simulink model "VCU_SW_1"  (R2023b)
settings: Solver=FixedStepDiscrete  StartTime=0.0  StopTime=inf  FixedStep=1e-2  RelTol=1e-3
PreLoadFcn:
  | RTWConfigurationCB('preloadfcn', bdroot);
InitFcn:
  | loadvar_ttc500
undefined symbols (not defined in the file): BrkPedalTypes, CabMovModeTypes, cFuseTempSensAcc_X, cFuseTempSensAcc_Y, cFuseTempSensVal_X, cFuseTempSensVal_Y, cTMSTempSensVal_X, cTMSTempSensVal_Y, cTransferCaseSpeedRatio, diag_state, DoorsPositionTypes, dP_filter_Y, DriverOccClassSystemTypes, ErrorValueTypes, fatal_error_callback, IO_ADC_NO_RANGE, LadderStatusTypes, pAnalogCabRotSensAcc, pAnalogCabRotSensMaxVolt, pAnalogCabRotSensMinVolt, pAnalogCabRotSensRange, pAnalogCabRotSensZeroVolt, pBrkActivePress, pCabTiltSensAcc, pCabTiltSensMaxCur, pCabTiltSensMinCur, pDistanceCorrection, pECANManual_BPNEnable, pECANManual_BPNEnabler_Flag, pFilterSensAccRes, pHDirMaxDiffFrq, pHDirSensHighLvl, pHDirSensLowLvl, pMainGearRatio, pMaxFilterSensRes, pMaxFirstPedalSensValue, pMaxFuseTempSensRes, pMaxPressLoss, pMaxPressSensCurrent, pMaxPressValue, pMaxPressValueHydMotAndPump, pMaxPressValueParkDrain, pMaxSecondPedalSensValue, pMaxTempSensVoltage, pMaxTempValue, pMaxTMSTempSensRes, pMinFilterSensRes, pMinFirstPedalSensValue, pMinFuseTempSensRes, pMinPressLoss, pMinPressSensCurrent, pMinPressValue, pMinSecondPedalSensValue, pMinTempSensVoltage, pMinTempValue, pMinTMSTempSensRes, pMotorRingTeethNum, pPedalSensAccuracyPct, pPedalSensAccuracyVolt, pPressLossTreshhold ... (+20)
libraries: TTlibrary x270, canmsglib x127, simulink x88
(part 4 of 19)

== system VCU_SW_1/InputLayer/InputInterfaces/PWDInput/GetPWD100msec ==
  function : TriggerPort  TriggerType=function-call  VariantControl=Variant
  Bus Selector : BusSelector  OutputSignals=pulse_samples_count
  Bus Selector1 : BusSelector  OutputSignals=pulse_samples_count
  Data Store Write : DataStoreWrite  DataStoreName=LogInputInterfaceData  DataStoreElements=LogInputInterfaceData.AI_1_Log.log_transPumpSpdSensSig2  IndexOptions=Index vector (dialog)  Indices=1  OutputSizes=1
  Data Store Write1 : DataStoreWrite  DataStoreName=InputInterfaceData  DataStoreElements=InputInterfaceData.PWD.transmHydMotSpdSensSig1  IndexOptions=Index vector (dialog)  Indices=1  OutputSizes=1
  Data Store Write10 : DataStoreWrite  DataStoreName=UDSStruct  DataStoreElements=UDSStruct.pin_transmHydMotSpdSensSig1  IndexOptions=Index vector (dialog)  Indices=1  OutputSizes=1
  Data Store Write11 : DataStoreWrite  DataStoreName=UDSStruct  DataStoreElements=UDSStruct.pin_transmHydMotSpdSensSig2  IndexOptions=Index vector (dialog)  Indices=1  OutputSizes=1
  Data Store Write12 : DataStoreWrite  DataStoreName=UDSStruct  DataStoreElements=UDSStruct.pin_transPumpSpdSensSig2  IndexOptions=Index vector (dialog)  Indices=1  OutputSizes=1
  Data Store Write13 : DataStoreWrite  DataStoreName=UDSStruct  DataStoreElements=UDSStruct.pin_transPumpSpdSensSig1  IndexOptions=Index vector (dialog)  Indices=1  OutputSizes=1
  Data Store Write2 : DataStoreWrite  DataStoreName=InputInterfaceData  DataStoreElements=InputInterfaceData.PWD.transmHydMotSpdSensSig2  IndexOptions=Index vector (dialog)  Indices=1  OutputSizes=1
  Data Store Write3 : DataStoreWrite  DataStoreName=InputInterfaceData  DataStoreElements=InputInterfaceData.PWD.transPumpSpdSensSig2  IndexOptions=Index vector (dialog)  Indices=1  OutputSizes=1
  Data Store Write4 : DataStoreWrite  DataStoreName=InputInterfaceData  DataStoreElements=InputInterfaceData.PWD.transPumpSpdSensSig1  IndexOptions=Index vector (dialog)  Indices=1  OutputSizes=1
  Data Store Write5 : DataStoreWrite  DataStoreName=LogInputInterfaceData  DataStoreElements=LogInputInterfaceData.AI_1_Log.log_transPumpSpdSensSig1  IndexOptions=Index vector (dialog)  Indices=1  OutputSizes=1
  Data Store Write6 : DataStoreWrite  DataStoreName=LogInputInterfaceData  DataStoreElements=LogInputInterfaceData.AI_2_Log.log_transmHydMotSpdSensSig1  IndexOptions=Index vector (dialog)  Indices=1  OutputSizes=1
  Data Store Write7 : DataStoreWrite  DataStoreName=LogInputInterfaceData  DataStoreElements=LogInputInterfaceData.AI_2_Log.log_transmHydMotSpdSensSig2  IndexOptions=Index vector (dialog)  Indices=1  OutputSizes=1
  Data Store Write8 : DataStoreWrite  DataStoreName=InputInterfaceData  DataStoreElements=InputInterfaceData.PWD.transmHydMotPulseSamples1  IndexOptions=Index vector (dialog)  Indices=1  OutputSizes=1
  Data Store Write9 : DataStoreWrite  DataStoreName=InputInterfaceData  DataStoreElements=InputInterfaceData.PWD.transmHydMotPulseSamples2  IndexOptions=Index vector (dialog)  Indices=1  OutputSizes=1
  Data Type Conversion : DataTypeConversion  OutDataTypeStr=uint16  SaturateOnIntegerOverflow=off  RndMeth=Floor
  Data Type Conversion1 : DataTypeConversion  OutDataTypeStr=uint16  SaturateOnIntegerOverflow=off  RndMeth=Floor
  Function Caller{,1..3} (4 alike) : FunctionCaller  FunctionPrototype=finalValue = convPWDData(rawValue,errorSts)  InputArgumentSpecifications=<Enter example>  OutputArgumentSpecifications=<Enter example>
  MATLAB Function8 : MATLAB Function  Commented=on  TreatAsAtomicUnit=on
  Terminator{,1..4,6,8..10,12} (10 alike) : Terminator
  TransPumpSpeedSensSig1 : TTlibrary/PWD/pwdComplexGet  timer_channel=IO_PWD_01  pulse_mode=IO_PWD_HIGH_TIME  freq_mode=IO_PWD_RISING_VAR  capture_count=4  pupd=IO_PWD_PD_10K  safety_conf=off  pwd_freq_val_lower=0  pwd_freq_val_upper=0  pwd_pulse_val_lower=0  pwd_pulse_val_upper=0  io_error=on  sample_time=-1
      settings: SourceProductName=TT control 500 series
  TransPumpSpeedSensSig2 : TTlibrary/PWD/pwdComplexGet  timer_channel=IO_PWD_03  pulse_mode=IO_PWD_HIGH_TIME  freq_mode=IO_PWD_RISING_VAR  capture_count=4  pupd=IO_PWD_PD_10K  safety_conf=off  pwd_freq_val_lower=0  pwd_freq_val_upper=0  pwd_pulse_val_lower=0  pwd_pulse_val_upper=0  io_error=on  sample_time=-1
      settings: SourceProductName=TT control 500 series
  TransmHydromotorSpeedAndPulseSig1 : TTlibrary/PWD/pwdComplexGet  timer_channel=IO_PWD_02  pulse_mode=IO_PWD_HIGH_TIME  freq_mode=IO_PWD_RISING_VAR  capture_count=4  pupd=IO_PWD_PD_10K  safety_conf=off  pwd_freq_val_lower=0  pwd_freq_val_upper=0  pwd_pulse_val_lower=0  pwd_pulse_val_upper=0  io_error=on  sample_time=-1
      settings: SourceProductName=TT control 500 series
  TransmHydromotorSpeedAndPulseSig2 : TTlibrary/PWD/pwdComplexGet  timer_channel=IO_PWD_04  pulse_mode=IO_PWD_HIGH_TIME  freq_mode=IO_PWD_RISING_VAR  capture_count=4  pupd=IO_PWD_PD_10K  safety_conf=off  pwd_freq_val_lower=0  pwd_freq_val_upper=0  pwd_pulse_val_lower=0  pwd_pulse_val_upper=0  io_error=on  sample_time=-1
      settings: SourceProductName=TT control 500 series
  wires:
  Data Type Conversion1/1 -> Data Store Write9/1
  TransmHydromotorSpeedAndPulseSig2/4 -> Bus Selector1/1  "io_pwd_04_samples"
  Bus Selector1/1 -> Data Type Conversion1/1  "<pulse_samples_count>"
  Data Type Conversion/1 -> Data Store Write8/1
  Bus Selector/1 -> Data Type Conversion/1  "<pulse_samples_count>"
  TransmHydromotorSpeedAndPulseSig1/4 -> Bus Selector/1  "io_pwd_02_samples"
  TransmHydromotorSpeedAndPulseSig2/1 -> Function Caller1/1  "io_pwd_04_freq_value"
  TransPumpSpeedSensSig2/1 -> Function Caller3/1  "io_pwd_03_freq_value"
  TransPumpSpeedSensSig1/1 -> Function Caller2/1  "io_pwd_01_freq_value"
  TransPumpSpeedSensSig2/4 -> Terminator10/1  "io_pwd_03_samples"
  TransPumpSpeedSensSig2/3 -> Terminator4/1  "io_pwd_03_pin_value"
  Function Caller/1 -> Data Store Write6/1, Data Store Write1/1
  TransPumpSpeedSensSig1/4 -> Terminator8/1  "io_pwd_01_samples"
  TransPumpSpeedSensSig2/2 -> Terminator9/1  "io_pwd_03_pw_value"
  TransmHydromotorSpeedAndPulseSig2/2 -> Terminator6/1  "io_pwd_04_pw_value"
  TransPumpSpeedSensSig2/5 -> Data Store Write13/1, Function Caller3/2  "io_pwd_03_error"
  Function Caller2/1 -> Data Store Write3/1, Data Store Write/1
  TransmHydromotorSpeedAndPulseSig1/5 -> Data Store Write10/1, Function Caller/2  "io_pwd_02_error"
  TransmHydromotorSpeedAndPulseSig1/1 -> Function Caller/1  "io_pwd_02_freq_value"
  TransmHydromotorSpeedAndPulseSig2/3 -> Terminator1/1  "io_pwd_04_pin_value"
  TransPumpSpeedSensSig1/2 -> Terminator3/1  "io_pwd_01_pw_value"
  TransPumpSpeedSensSig1/3 -> Terminator2/1  "io_pwd_01_pin_value"
  TransPumpSpeedSensSig1/5 -> Function Caller2/2, Data Store Write12/1  "io_pwd_01_error"
  Function Caller3/1 -> Data Store Write4/1, Data Store Write5/1
  Function Caller1/1 -> Data Store Write7/1, Data Store Write2/1
  TransmHydromotorSpeedAndPulseSig1/3 -> Terminator/1  "io_pwd_02_pin_value"
  TransmHydromotorSpeedAndPulseSig1/2 -> Terminator12/1  "io_pwd_02_pw_value"
  TransmHydromotorSpeedAndPulseSig2/5 -> Data Store Write11/1, Function Caller1/2  "io_pwd_04_error"

== system VCU_SW_1/InputLayer/InputInterfaces/PWDInput/GetPWD10msec ==
  function : TriggerPort  TriggerType=function-call  VariantControl=Variant

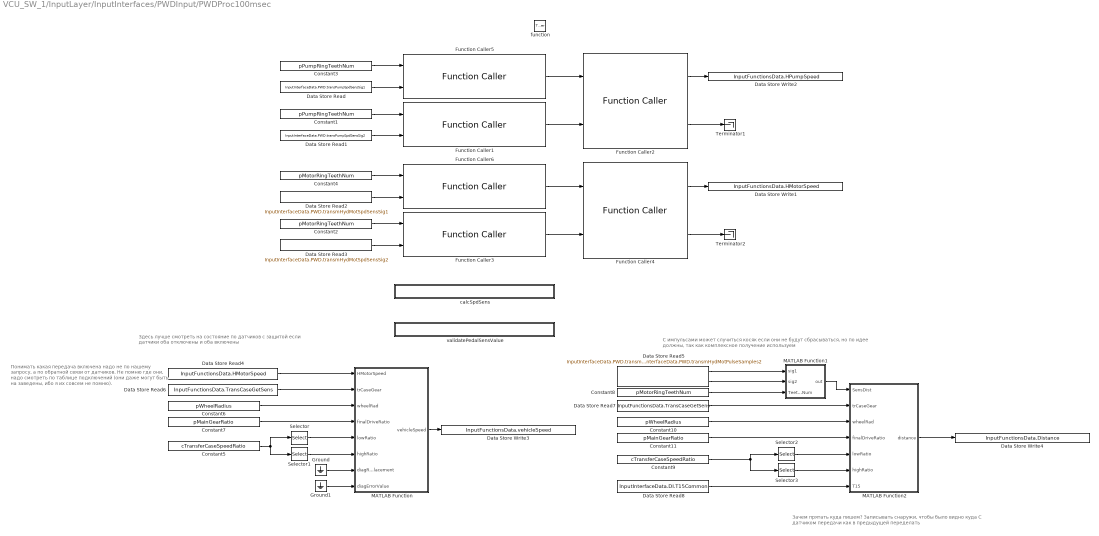
== system VCU_SW_1/InputLayer/InputInterfaces/PWDInput/PWDProc100msec ==
  note: Понимать какая передача включена надо не по нашему запросу, а по обратной связи от датчиков.
      | Не помню где они, надо смотреть по таблице подключений (они даже могут быть на заведены, ибо я их совсем не помню).
  note: С импульсами может случиться косяк если они не будут сбрасываться, но по идее должны, так как комплексное получение используем
  note: Зачем прятать куда пишем? Записывать снаружи, чтобы было видно куда
      | С датчиком передачи как в предыдущей переделать
  note: Здесь лучше смотреть на состояние по датчиков
      | с защитой если датчики оба отключены и оба включены
  function : TriggerPort  TriggerType=function-call  VariantControl=Variant
  Constant1 : Constant  Value=pPumpRingTeethNum
  Constant10 : Constant  Value=pWheelRadius
  Constant11 : Constant  Value=pMainGearRatio
  Constant2 : Constant  Value=pMotorRingTeethNum
  Constant3 : Constant  Value=pPumpRingTeethNum
  Constant4 : Constant  Value=pMotorRingTeethNum
  Constant5 : Constant  Value=cTransferCaseSpeedRatio
  Constant6 : Constant  Value=pWheelRadius
  Constant7 : Constant  Value=pMainGearRatio
  Constant8 : Constant  Value=pMotorRingTeethNum
  Constant9 : Constant  Value=cTransferCaseSpeedRatio
  Data Store Read : DataStoreRead  DataStoreName=InputInterfaceData  DataStoreElements=InputInterfaceData.PWD.transPumpSpdSensSig1  IndexOptions=Index vector (dialog)  Indices=1  OutputSizes=1
  Data Store Read1 : DataStoreRead  DataStoreName=InputInterfaceData  DataStoreElements=InputInterfaceData.PWD.transPumpSpdSensSig2  IndexOptions=Index vector (dialog)  Indices=1  OutputSizes=1
  Data Store Read2 : DataStoreRead  DataStoreName=InputInterfaceData  DataStoreElements=InputInterfaceData.PWD.transmHydMotSpdSensSig1  IndexOptions=Index vector (dialog)  Indices=1  OutputSizes=1
  Data Store Read3 : DataStoreRead  DataStoreName=InputInterfaceData  DataStoreElements=InputInterfaceData.PWD.transmHydMotSpdSensSig2  IndexOptions=Index vector (dialog)  Indices=1  OutputSizes=1
  Data Store Read4 : DataStoreRead  DataStoreName=InputFunctionsData  DataStoreElements=InputFunctionsData.HMotorSpeed  IndexOptions=Index vector (dialog)  Indices=1  OutputSizes=1
  Data Store Read5 : DataStoreRead  DataStoreName=InputInterfaceData  DataStoreElements=InputInterfaceData.PWD.transmHydMotPulseSamples1#InputInterfaceData.PWD.transmHydMotPulseSamples2  IndexOptions=Index vector (dialog)  Indices=1  OutputSizes=1
  Data Store Read6 : DataStoreRead  DataStoreName=InputFunctionsData  DataStoreElements=InputFunctionsData.TransCaseGetSens  IndexOptions=Index vector (dialog)  Indices=1  OutputSizes=1
  Data Store Read7 : DataStoreRead  DataStoreName=InputFunctionsData  DataStoreElements=InputFunctionsData.TransCaseGetSens  IndexOptions=Index vector (dialog)  Indices=1  OutputSizes=1
  Data Store Read8 : DataStoreRead  DataStoreName=InputInterfaceData  DataStoreElements=InputInterfaceData.DI.T15Common  IndexOptions=Index vector (dialog)  Indices=1  OutputSizes=1
  Data Store Write1 : DataStoreWrite  DataStoreName=InputFunctionsData  DataStoreElements=InputFunctionsData.HMotorSpeed  IndexOptions=Index vector (dialog)  Indices=1  OutputSizes=1
  Data Store Write2 : DataStoreWrite  DataStoreName=InputFunctionsData  DataStoreElements=InputFunctionsData.HPumpSpeed  IndexOptions=Index vector (dialog)  Indices=1  OutputSizes=1
  Data Store Write3 : DataStoreWrite  DataStoreName=InputFunctionsData  DataStoreElements=InputFunctionsData.vehicleSpeed  IndexOptions=Index vector (dialog)  Indices=1  OutputSizes=1
  Data Store Write4 : DataStoreWrite  DataStoreName=InputFunctionsData  DataStoreElements=InputFunctionsData.Distance  IndexOptions=Index vector (dialog)  Indices=1  OutputSizes=1
  Function Caller{1,3,5..6} (4 alike) : FunctionCaller  FunctionPrototype=SpdValue = calcSpdSensValue(teethNum,sensFreq)  InputArgumentSpecifications=<Enter example>  OutputArgumentSpecifications=<Enter example>
  Function Caller2 : FunctionCaller  FunctionPrototype=[SpdVal,errorSts] = validateSpdSensValue(fstValue,secValue)  InputArgumentSpecifications=<Enter example>  OutputArgumentSpecifications=<Enter example>
  Function Caller4 : FunctionCaller  FunctionPrototype=[SpdVal,errorSts] = validateSpdSensValue(fstValue,secValue)  InputArgumentSpecifications=<Enter example>  OutputArgumentSpecifications=<Enter example>
  Ground : Ground
  Ground1 : Ground
  MATLAB Function : MATLAB Function  TreatAsAtomicUnit=on
  MATLAB Function1 : MATLAB Function  TreatAsAtomicUnit=on
  MATLAB Function2 : MATLAB Function  TreatAsAtomicUnit=on
  Selector : Selector  InputPortWidth=2  IndexOptions=Index vector (dialog)  Indices=2  OutputSizes=1
  Selector1 : Selector  InputPortWidth=2  IndexOptions=Index vector (dialog)  Indices=1  OutputSizes=1
  Selector2 : Selector  InputPortWidth=2  IndexOptions=Index vector (dialog)  Indices=2  OutputSizes=1
  Selector3 : Selector  InputPortWidth=2  IndexOptions=Index vector (dialog)  Indices=1  OutputSizes=1
  Terminator1 : Terminator
  Terminator2 : Terminator
  calcSpdSens : Subsystem  TreatAsAtomicUnit=on
  validatePedalSensValue : Subsystem  TreatAsAtomicUnit=on
  wires:
  Data Store Read8/1 -> MATLAB Function2/7(T15)
  Data Store Read7/1 -> MATLAB Function2/2(trCaseGear)
  MATLAB Function1/1(out) -> MATLAB Function2/1(SensDist)
  Constant10/1 -> MATLAB Function2/3(wheelRad)
  Constant11/1 -> MATLAB Function2/4(finalDriveRatio)
  Selector3/1 -> MATLAB Function2/6(highRatio)
  Selector2/1 -> MATLAB Function2/5(lowRatio)
  Constant9/1 -> Selector2/1, Selector3/1
  Constant8/1 -> MATLAB Function1/3(TeethNum)
  Data Store Read5/2 -> MATLAB Function1/2(sig2)
  Data Store Read5/1 -> MATLAB Function1/1(sig1)
  Data Store Read1/1 -> Function Caller1/2
  Data Store Read/1 -> Function Caller5/2
  Function Caller3/1 -> Function Caller4/2
  Function Caller1/1 -> Function Caller2/2
  Function Caller4/1 -> Data Store Write1/1
  Constant1/1 -> Function Caller1/1
  Constant2/1 -> Function Caller3/1
  Constant4/1 -> Function Caller6/1
  Data Store Read2/1 -> Function Caller6/2
  Data Store Read3/1 -> Function Caller3/2
  Constant3/1 -> Function Caller5/1
  Function Caller2/1 -> Data Store Write2/1
  Function Caller4/2 -> Terminator2/1
  Function Caller6/1 -> Function Caller4/1
  Function Caller5/1 -> Function Caller2/1
  Function Caller2/2 -> Terminator1/1
  MATLAB Function2/1(distance) -> Data Store Write4/1
  Constant5/1 -> Selector/1, Selector1/1
  Constant7/1 -> MATLAB Function/4(finalDriveRatio)
  Data Store Read6/1 -> MATLAB Function/2(trCaseGear)
  Selector1/1 -> MATLAB Function/6(highRatio)
  Selector/1 -> MATLAB Function/5(lowRatio)
  Data Store Read4/1 -> MATLAB Function/1(HMotorSpeed)
  Ground1/1 -> MATLAB Function/8(diagErrorValue)
  Constant6/1 -> MATLAB Function/3(wheelRad)
  Ground/1 -> MATLAB Function/7(diagReplacement)
  MATLAB Function/1(vehicleSpeed) -> Data Store Write3/1

== system VCU_SW_1/InputLayer/InputInterfaces/PWMCurrentInput/GetPWMCur1000msec ==
  function : TriggerPort  TriggerType=function-call  VariantControl=Variant

== system VCU_SW_1/InputLayer/InputInterfaces/PWMCurrentInput/GetPWMCur100msec ==
  function : TriggerPort  TriggerType=function-call  VariantControl=Variant

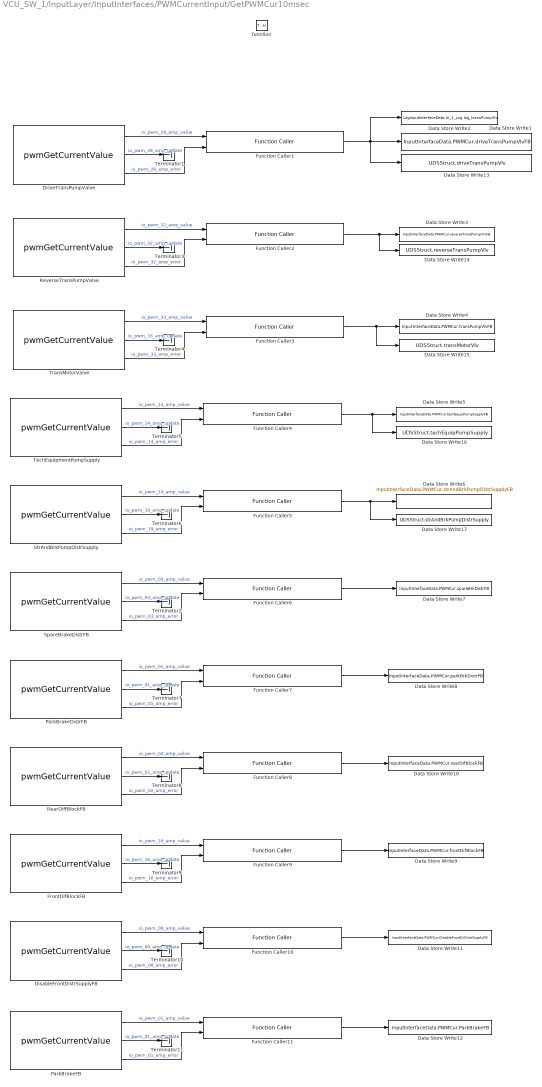
== system VCU_SW_1/InputLayer/InputInterfaces/PWMCurrentInput/GetPWMCur10msec ==
  function : TriggerPort  TriggerType=function-call  VariantControl=Variant
  Data Store Write1 : DataStoreWrite  DataStoreName=InputInterfaceData  DataStoreElements=InputInterfaceData.PWMCur.driveTransPumpVlvFB  IndexOptions=Index vector (dialog)  Indices=1  OutputSizes=1
  Data Store Write10 : DataStoreWrite  DataStoreName=InputInterfaceData  DataStoreElements=InputInterfaceData.PWMCur.rearDifBlockFB  IndexOptions=Index vector (dialog)  Indices=1  OutputSizes=1
  Data Store Write11 : DataStoreWrite  DataStoreName=InputInterfaceData  DataStoreElements=InputInterfaceData.PWMCur.DisableFrontDrDistrSupplyFB  IndexOptions=Index vector (dialog)  Indices=1  OutputSizes=1
  Data Store Write12 : DataStoreWrite  DataStoreName=InputInterfaceData  DataStoreElements=InputInterfaceData.PWMCur.ParkBrakeFB  IndexOptions=Index vector (dialog)  Indices=1  OutputSizes=1
  Data Store Write13 : DataStoreWrite  DataStoreName=UDSStruct  DataStoreElements=UDSStruct.driveTransPumpVlv  IndexOptions=Index vector (dialog)  Indices=1  OutputSizes=1
  Data Store Write14 : DataStoreWrite  DataStoreName=UDSStruct  DataStoreElements=UDSStruct.reverseTransPumpVlv  IndexOptions=Index vector (dialog)  Indices=1  OutputSizes=1
  Data Store Write15 : DataStoreWrite  DataStoreName=UDSStruct  DataStoreElements=UDSStruct.transMotorVlv  IndexOptions=Index vector (dialog)  Indices=1  OutputSizes=1
  Data Store Write16 : DataStoreWrite  DataStoreName=UDSStruct  DataStoreElements=UDSStruct.techEquipPumpSupply  IndexOptions=Index vector (dialog)  Indices=1  OutputSizes=1
  Data Store Write17 : DataStoreWrite  DataStoreName=UDSStruct  DataStoreElements=UDSStruct.strAndBrkPumpDistrSupply  IndexOptions=Index vector (dialog)  Indices=1  OutputSizes=1
  Data Store Write2 : DataStoreWrite  DataStoreName=LogInputInterfaceData  DataStoreElements=LogInputInterfaceData.AI_1_Log.log_transPumpVlv  IndexOptions=Index vector (dialog)  Indices=1  OutputSizes=1
  Data Store Write3 : DataStoreWrite  DataStoreName=InputInterfaceData  DataStoreElements=InputInterfaceData.PWMCur.reverseTransPumpVlvFB  IndexOptions=Index vector (dialog)  Indices=1  OutputSizes=1
  Data Store Write4 : DataStoreWrite  DataStoreName=InputInterfaceData  DataStoreElements=InputInterfaceData.PWMCur.transPumpVlvFB  IndexOptions=Index vector (dialog)  Indices=1  OutputSizes=1
  Data Store Write5 : DataStoreWrite  DataStoreName=InputInterfaceData  DataStoreElements=InputInterfaceData.PWMCur.techEquipPumpSupplyFB  IndexOptions=Index vector (dialog)  Indices=1  OutputSizes=1
  Data Store Write6 : DataStoreWrite  DataStoreName=InputInterfaceData  DataStoreElements=InputInterfaceData.PWMCur.strAndBrkPumpDistrSupplyFB  IndexOptions=Index vector (dialog)  Indices=1  OutputSizes=1
  Data Store Write7 : DataStoreWrite  DataStoreName=InputInterfaceData  DataStoreElements=InputInterfaceData.PWMCur.spareBrkDistrFB  IndexOptions=Index vector (dialog)  Indices=1  OutputSizes=1
  Data Store Write8 : DataStoreWrite  DataStoreName=InputInterfaceData  DataStoreElements=InputInterfaceData.PWMCur.parkBrkDistrFB  IndexOptions=Index vector (dialog)  Indices=1  OutputSizes=1
  Data Store Write9 : DataStoreWrite  DataStoreName=InputInterfaceData  DataStoreElements=InputInterfaceData.PWMCur.frontDifBlockFB  IndexOptions=Index vector (dialog)  Indices=1  OutputSizes=1
  DisableFrontDistrSupplyFB : TTlibrary/PWM /pwmGetCurrentValue  pwm_channel=IO_PWM_09  io_error=on  sample_time=-1
      settings: SourceProductName=TT control 500 series
  DriveTransPumpValve : TTlibrary/PWM /pwmGetCurrentValue  pwm_channel=IO_PWM_28  io_error=on  sample_time=-1
      settings: SourceProductName=TT control 500 series
  FrontDifBlockFB : TTlibrary/PWM /pwmGetCurrentValue  pwm_channel=IO_PWM_16  io_error=on  sample_time=-1
      settings: SourceProductName=TT control 500 series
  Function Caller{1..11} (11 alike) : FunctionCaller  FunctionPrototype=finalValue = convPWMCurrData(rawValue,errorSts)  InputArgumentSpecifications=<Enter example>  OutputArgumentSpecifications=<Enter example>
  ParkBrakeDistrFB : TTlibrary/PWM /pwmGetCurrentValue  pwm_channel=IO_PWM_01  io_error=on  sample_time=-1
      settings: SourceProductName=TT control 500 series
  ParkBrakeFB : TTlibrary/PWM /pwmGetCurrentValue  pwm_channel=IO_PWM_01  io_error=on  sample_time=-1
      settings: SourceProductName=TT control 500 series
  RearDiffBlockFB : TTlibrary/PWM /pwmGetCurrentValue  pwm_channel=IO_PWM_02  io_error=on  sample_time=-1
      settings: SourceProductName=TT control 500 series
  ReverseTransPumpValve : TTlibrary/PWM /pwmGetCurrentValue  pwm_channel=IO_PWM_32  io_error=on  sample_time=-1
      settings: SourceProductName=TT control 500 series
  SpareBrakeDistrFB : TTlibrary/PWM /pwmGetCurrentValue  pwm_channel=IO_PWM_03  io_error=on  sample_time=-1
      settings: SourceProductName=TT control 500 series
  StrAndBrkPumpDistrSupply : TTlibrary/PWM /pwmGetCurrentValue  pwm_channel=IO_PWM_19  io_error=on  sample_time=-1
      settings: SourceProductName=TT control 500 series
  TechEquipmentPumpSupply : TTlibrary/PWM /pwmGetCurrentValue  pwm_channel=IO_PWM_14  io_error=on  sample_time=-1
      settings: SourceProductName=TT control 500 series
  Terminator{1..11} (11 alike) : Terminator
  TransMotorValve : TTlibrary/PWM /pwmGetCurrentValue  pwm_channel=IO_PWM_33  io_error=on  sample_time=-1
      settings: SourceProductName=TT control 500 series
  wires:
  Function Caller7/1 -> Data Store Write8/1
  ParkBrakeDistrFB/2 -> Terminator7/1  "io_pwm_01_amp_update"
  ParkBrakeDistrFB/1 -> Function Caller7/1  "io_pwm_01_amp_value"
  ParkBrakeDistrFB/3 -> Function Caller7/2  "io_pwm_01_amp_error"
  SpareBrakeDistrFB/3 -> Function Caller6/2  "io_pwm_03_amp_error"
  SpareBrakeDistrFB/1 -> Function Caller6/1  "io_pwm_03_amp_value"
  SpareBrakeDistrFB/2 -> Terminator2/1  "io_pwm_03_amp_update"
  Function Caller6/1 -> Data Store Write7/1
  Function Caller1/1 -> Data Store Write13/1, Data Store Write1/1, Data Store Write2/1
  StrAndBrkPumpDistrSupply/3 -> Function Caller5/2  "io_pwm_19_amp_error"
  Function Caller5/1 -> Data Store Write17/1, Data Store Write6/1
  StrAndBrkPumpDistrSupply/1 -> Function Caller5/1  "io_pwm_19_amp_value"
  StrAndBrkPumpDistrSupply/2 -> Terminator6/1  "io_pwm_19_amp_update"
  TechEquipmentPumpSupply/3 -> Function Caller4/2  "io_pwm_14_amp_error"
  Function Caller4/1 -> Data Store Write16/1, Data Store Write5/1
  TechEquipmentPumpSupply/1 -> Function Caller4/1  "io_pwm_14_amp_value"
  TechEquipmentPumpSupply/2 -> Terminator5/1  "io_pwm_14_amp_update"
  TransMotorValve/3 -> Function Caller3/2  "io_pwm_33_amp_error"
  Function Caller3/1 -> Data Store Write15/1, Data Store Write4/1
  TransMotorValve/1 -> Function Caller3/1  "io_pwm_33_amp_value"
  TransMotorValve/2 -> Terminator4/1  "io_pwm_33_amp_update"
  ReverseTransPumpValve/3 -> Function Caller2/2  "io_pwm_32_amp_error"
  Function Caller2/1 -> Data Store Write14/1, Data Store Write3/1
  ReverseTransPumpValve/1 -> Function Caller2/1  "io_pwm_32_amp_value"
  ReverseTransPumpValve/2 -> Terminator3/1  "io_pwm_32_amp_update"
  DriveTransPumpValve/3 -> Function Caller1/2  "io_pwm_28_amp_error"
  DriveTransPumpValve/1 -> Function Caller1/1  "io_pwm_28_amp_value"
  DriveTransPumpValve/2 -> Terminator1/1  "io_pwm_28_amp_update"
  RearDiffBlockFB/2 -> Terminator8/1  "io_pwm_02_amp_update"
  RearDiffBlockFB/3 -> Function Caller8/2  "io_pwm_02_amp_error"
  FrontDifBlockFB/3 -> Function Caller9/2  "io_pwm_16_amp_error"
  FrontDifBlockFB/1 -> Function Caller9/1  "io_pwm_16_amp_value"
  FrontDifBlockFB/2 -> Terminator9/1  "io_pwm_16_amp_update"
  RearDiffBlockFB/1 -> Function Caller8/1  "io_pwm_02_amp_value"
  Function Caller8/1 -> Data Store Write10/1
  Function Caller9/1 -> Data Store Write9/1
  Function Caller10/1 -> Data Store Write11/1
  DisableFrontDistrSupplyFB/2 -> Terminator10/1  "io_pwm_09_amp_update"
  DisableFrontDistrSupplyFB/1 -> Function Caller10/1  "io_pwm_09_amp_value"
  DisableFrontDistrSupplyFB/3 -> Function Caller10/2  "io_pwm_09_amp_error"
  ParkBrakeFB/3 -> Function Caller11/2  "io_pwm_01_amp_error"
  ParkBrakeFB/1 -> Function Caller11/1  "io_pwm_01_amp_value"
  ParkBrakeFB/2 -> Terminator11/1  "io_pwm_01_amp_update"
  Function Caller11/1 -> Data Store Write12/1

== system VCU_SW_1/InputLayer/InputInterfaces/PWMCurrentInput/PWMCur10msecProc ==
  function : TriggerPort  TriggerType=function-call  VariantControl=Variant
  Constant12 : Constant  Value=pValveActiveCur
  Data Store Read : DataStoreRead  DataStoreName=InputInterfaceData  DataStoreElements=InputInterfaceData.PWMCur.DisableFrontDrDistrSupplyFB  IndexOptions=Index vector (dialog)  Indices=1  OutputSizes=1
  Data Store Read1 : DataStoreRead  DataStoreName=InputInterfaceData  DataStoreElements=InputInterfaceData.PWMCur.parkBrkDistrFB  IndexOptions=Index vector (dialog)  Indices=1  OutputSizes=1
  Data Store Read12 : DataStoreRead  DataStoreName=InputInterfaceData  DataStoreElements=InputInterfaceData.PWMCur.spareBrkDistrFB  IndexOptions=Index vector (dialog)  Indices=1  OutputSizes=1
  Data Store Read2 : DataStoreRead  DataStoreName=InputInterfaceData  DataStoreElements=InputInterfaceData.PWMCur.frontDifBlockFB  IndexOptions=Index vector (dialog)  Indices=1  OutputSizes=1
  Data Store Read3 : DataStoreRead  DataStoreName=InputInterfaceData  DataStoreElements=InputInterfaceData.PWMCur.rearDifBlockFB  IndexOptions=Index vector (dialog)  Indices=1  OutputSizes=1
  Data Store Write : DataStoreWrite  DataStoreName=InputFunctionsData  DataStoreElements=InputFunctionsData.frontDifBlockFB  IndexOptions=Index vector (dialog)  Indices=1  OutputSizes=1
  Data Store Write1 : DataStoreWrite  DataStoreName=InputFunctionsData  DataStoreElements=InputFunctionsData.spareBrkDistrFB  IndexOptions=Index vector (dialog)  Indices=1  OutputSizes=1
  Data Store Write2 : DataStoreWrite  DataStoreName=InputFunctionsData  DataStoreElements=InputFunctionsData.parkBrkDistrFB  IndexOptions=Index vector (dialog)  Indices=1  OutputSizes=1
  Data Store Write3 : DataStoreWrite  DataStoreName=InputFunctionsData  DataStoreElements=InputFunctionsData.rearDifBlockFB  IndexOptions=Index vector (dialog)  Indices=1  OutputSizes=1
  Data Store Write4 : DataStoreWrite  DataStoreName=InputFunctionsData  DataStoreElements=InputFunctionsData.DisableFrontDrDistrSupplyFB  IndexOptions=Index vector (dialog)  Indices=1  OutputSizes=1
  Data Store Write5 : DataStoreWrite  DataStoreName=InputFunctionsData  DataStoreElements=InputFunctionsData.parkBrakeFB  IndexOptions=Index vector (dialog)  Indices=1  OutputSizes=1
  Function Caller{,1..4} (5 alike) : FunctionCaller  FunctionPrototype=stt = ValveCurFBproc(pValveActiveCur,curFB)  InputArgumentSpecifications=<Enter example>  OutputArgumentSpecifications=<Enter example>
  MATLAB Function2 : MATLAB Function  TreatAsAtomicUnit=on
  Simulink Function : Subsystem  TreatAsAtomicUnit=on
  wires:
  Constant12/1 -> Function Caller1/1, Function Caller/1, Function Caller2/1, Function Caller3/1, Function Caller4/1
  Function Caller4/1 -> Data Store Write4/1
  Data Store Read/1 -> Function Caller4/2
  Data Store Read3/1 -> Function Caller3/2
  Data Store Read2/1 -> Function Caller2/2
  Function Caller3/1 -> Data Store Write3/1
  Function Caller2/1 -> Data Store Write/1
  Function Caller1/1 -> Data Store Write1/1
  Data Store Read1/1 -> Function Caller/2
  Function Caller/1 -> MATLAB Function2/1(sttRaw), Data Store Write2/1
  Data Store Read12/1 -> Function Caller1/2
  MATLAB Function2/1(sttInv) -> Data Store Write5/1

== system VCU_SW_1/InputLayer/InputNetwork/InputCCAN/CCAN100msecProc1 ==
  function : TriggerPort  TriggerType=function-call  VariantControl=Variant
  CabMov buttons processing : Subsystem  TreatAsAtomicUnit=on
  InputTransSelect : Subsystem  TreatAsAtomicUnit=on
  JoystickRot : Subsystem  TreatAsAtomicUnit=on

== system VCU_SW_1/InputLayer/InputNetwork/InputCCAN/CCAN10msecProc  ==
  function : TriggerPort  TriggerType=function-call  VariantControl=Variant

== system VCU_SW_1/InputLayer/InputNetwork/InputCCAN/GetCCAN1000msec ==
  function : TriggerPort  TriggerType=function-call  VariantControl=Variant
  DD : Subsystem
  "Fuel Heater Data " : Subsystem
  LCMD : Subsystem
  LD : Subsystem
  OCSI : Subsystem
  VF : Subsystem

== system VCU_SW_1/InputLayer/InputNetwork/InputCCAN/GetCCAN100msec ==
  note: КОСТЫЛЬ
  note: Вот тут тоже с типом данных матлаб функци брехня, посмотреть везде
  function : TriggerPort  TriggerType=function-call  VariantControl=Variant
  AUX_VLV_EST_CABIN : Subsystem
  BJM1 : Subsystem
  BJM2 : Subsystem
  CM1 : Subsystem
  CM3 : Subsystem
  CabinAuxiliaryStatus : Subsystem
  DC1 : Subsystem
  "Fan Rotation Direction Control " : Subsystem
  "Fan Rotation Direction Status " : Subsystem
  FuelTankAndFrameLock : Subsystem
  "Instrument Cluster Status " : Subsystem
  Left Big Pan Cmd : Subsystem
  Left Small Pan Cmd : Subsystem
  "OWW Status " : Subsystem
  PTO : Subsystem
  "Remote Brake Command " : Subsystem
  Right Small Pan Cmd : Subsystem
  TC1 : Subsystem

== system VCU_SW_1/InputLayer/InputNetwork/InputCCAN/GetCCAN10msec ==
  function : TriggerPort  TriggerType=function-call  VariantControl=Variant
  CAN_Unpack_PLC_StateM : canmsglib/CAN Unpack  Commented=on  MsgList=(none)  MsgName=PLC_StateM  MsgIDType=Extended (29-bit identifier)  MsgIdentifier=419388800  MsgLength=5  SignalInfo={ 'PLC_V2G_StateM_SM9MesState', '16', '8', 'LE', 'unsigned', 'Standard', '0', '1', '0', '0', '255'; 'PLC_V2G_StateM_SM9Status', '24', '8', 'LE', 'unsigned', 'Standard', '0', '1', '0', '0', '255' }  IDPort=off  TimestampPort=off  ErrorPort=off  RemotePort=off  LengthPort=off  StatusPort=off  ApplyMinMax=off
  DataStoreWrite_PLC_StateM : DataStoreWrite  Commented=on  DataStoreName=InputNetworkData  DataStoreElements=InputNetworkData.ECAN.PLC.PLC_V2G_StateM_SM9MesState#InputNetworkData.ECAN.PLC.PLC_V2G_StateM_SM9Status  IndexOptions=Index vector (dialog)  Indices=1  OutputSizes=1
  Terminator : Terminator  Commented=on
  read_message_PLC_StateM : TTlibrary/CAN/read_message_name  Commented=on  channel=IO_CAN_CHANNEL_1  id_format=IO_CAN_EXT_FRAME  get_msg_info=off  message_names=there is no CAN Unpack blocks  message_info=|  id=419388800  ac_mask=536870911  retranslation=off  io_error=on  sample_time=-1
      | Message Name: PLC_StateM
      |  Message ID Type: Extended (29-bit identifier)
      |  Message ID: 419388800
      settings: SourceProductName=TT control 500 series
  wires:
  read_message_PLC_StateM/1 -> CAN_Unpack_PLC_StateM/1  "msg_419388800"
  read_message_PLC_StateM/2 -> Terminator/1  "handler_err_419388800"
  CAN_Unpack_PLC_StateM/1 -> DataStoreWrite_PLC_StateM/1
  CAN_Unpack_PLC_StateM/2 -> DataStoreWrite_PLC_StateM/2

== system VCU_SW_1/InputLayer/InputNetwork/InputCCAN/GetCCAN200msec ==
  function : TriggerPort  TriggerType=function-call  VariantControl=Variant
  OWW : Subsystem

== system VCU_SW_1/InputLayer/InputNetwork/InputCCAN/GetCCAN500msec ==
  function : TriggerPort  TriggerType=function-call  VariantControl=Variant
  EAC1 : Subsystem

== system VCU_SW_1/InputLayer/InputNetwork/InputDiagCAN/GetDiagCAN10msec ==
  function : TriggerPort  TriggerType=function-call  VariantControl=Variant
  Data Store Write : DataStoreWrite  DataStoreName=UDSStruct  DataStoreElements=UDSStruct.readUDSmsgFlag  IndexOptions=Index vector (dialog)  Indices=1  OutputSizes=1
  MATLAB Function : MATLAB Function  TreatAsAtomicUnit=on
  Simulink Function : Subsystem  TreatAsAtomicUnit=on
  Simulink Function1 : Subsystem  TreatAsAtomicUnit=on
  Simulink Function2 : Subsystem  TreatAsAtomicUnit=on
  wires:
  MATLAB Function/1(ReadUDSmsgFlag) -> Data Store Write/1

== system VCU_SW_1/InputLayer/InputNetwork/InputDiagCAN/GetDiagCAN10msec1 ==
  function : TriggerPort  TriggerType=function-call  VariantControl=Variant
  MATLAB Function : MATLAB Function  TreatAsAtomicUnit=on
  Simulink Function1 : Subsystem  TreatAsAtomicUnit=on
  Simulink Function2 : Subsystem  TreatAsAtomicUnit=on

== system VCU_SW_1/InputLayer/InputNetwork/InputEngCAN/GetEngCAN1000msec ==
  function : TriggerPort  TriggerType=function-call  VariantControl=Variant
  CANUnpack_ECU_DLCC1 : canmsglib/CAN Unpack  MsgList=(none)  MsgName=ECU_DLCC1  MsgIDType=Extended (29-bit identifier)  MsgIdentifier=419235584  MsgLength=8  SignalInfo={ 'ECU_DLCC1_EngAirFiltRestrLampCmd', '22', '2', 'LE', 'unsigned', 'Standard', '0', '1', '0', '0', '3'; 'ECU_DLCC1_EngAmberWarnLampCmd', '2', '2', 'LE', 'unsigned', 'Standard', '0', '1', '0', '0', '3'; 'ECU_DLCC1_EngCoolLevLowLampCmd', '16', '2', 'LE', 'unsigned', 'Standard', '0', '1', '0', '0', '3'; 'ECU_DLCC1_EngCoolTempHiLampCmd', '14', '2', 'LE', 'unsigned', 'Standard', '0', '1', '0', '0', '3'; 'ECU_DLCC1_EngOilPressLowLampCmd', '12', '2', 'LE', 'unsigned', 'Standard', '0', '1', '0', '0', '3'; 'ECU_DLCC1_EngProtLampCmd', '0', '2', 'LE', 'unsigned', 'Standard', '0', '1', '0', '0', '3'; 'ECU_DLCC1_EngRedStopLampCmd', '4', '2', 'LE', 'unsigned', 'Standard', '0', '1', '0', '0', '3' }  IDPort=off  TimestampPort=off  ErrorPort=off  RemotePort=off  LengthPort=off  StatusPort=off  ApplyMinMax=off
  CANUnpack_ECU_ET1 : canmsglib/CAN Unpack  MsgList=(none)  MsgName=ECU_ET1  MsgIDType=Extended (29-bit identifier)  MsgIdentifier=419360256  MsgLength=8  SignalInfo={ 'ECU_ET1_EngCoolTemp', '0', '8', 'LE', 'unsigned', 'Standard', '0', '1', '-40', '-40', '210'; 'ECU_ET1_EngFuelTemp1', '8', '8', 'LE', 'unsigned', 'Standard', '0', '1', '-40', '-40', '210'; 'ECU_ET1_EngIntThOp', '56', '8', 'LE', 'unsigned', 'Standard', '0', '0.4', '0', '0', '100'; 'ECU_ET1_EngInterTemp', '48', '8', 'LE', 'unsigned', 'Standard', '0', '1', '-40', '-40', '210'; 'ECU_ET1_EngOilTemp1', '16', '16', 'LE', 'unsigned', 'Standard', '0', '0.03125', '-273', '-273', '1734.9688'; 'ECU_ET1_EngTurbOilTemp', '32', '16', 'LE', 'unsigned', 'Standard', '0', '0.03125', '-273', '-273', '1734.9688' }  IDPort=off  TimestampPort=off  ErrorPort=off  RemotePort=off  LengthPort=off  StatusPort=off  ApplyMinMax=off
  CANUnpack_ECU_ET2 : canmsglib/CAN Unpack  MsgList=(none)  MsgName=ECU_ET2  MsgIDType=Extended (29-bit identifier)  MsgIdentifier=419341312  MsgLength=8  SignalInfo={ 'ECU_ET2_EngECUTemp', '16', '16', 'LE', 'unsigned', 'Standard', '0', '0.03125', '-273', '-273', '1734.9688'; 'ECU_ET2_EngExGasRec1T', '48', '16', 'LE', 'unsigned', 'Standard', '0', '0.03125', '-273', '-273', '1734.9688'; 'ECU_ET2_EngExhGasRec1DP', '32', '16', 'LE', 'unsigned', 'Standard', '0', '0.0078125', '-250', '-250', '251.99'; 'ECU_ET2_EngOilTemp2', '0', '16', 'LE', 'unsigned', 'Standard', '0', '0.03125', '-273', '-273', '1734.9688' }  IDPort=off  TimestampPort=off  ErrorPort=off  RemotePort=off  LengthPort=off  StatusPort=off  ApplyMinMax=off
  CANUnpack_ECU_ET3 : canmsglib/CAN Unpack  MsgList=(none)  MsgName=ECU_THO  MsgIDType=Extended (29-bit identifier)  MsgIdentifier=419357952  MsgLength=8  SignalInfo={ 'EngTotalHours', '0', '32', 'LE', 'signed', 'Standard', '0', '0.05', '0', '0', '210554060.75' }  IDPort=off  TimestampPort=off  ErrorPort=off  RemotePort=off  LengthPort=off  StatusPort=off  ApplyMinMax=off
  CANUnpack_ECU_SHUTDN : canmsglib/CAN Unpack  MsgList=(none)  MsgName=ECU_SHUTDN  MsgIDType=Extended (29-bit identifier)  MsgIdentifier=419357696  MsgLength=8  SignalInfo={ 'ECU_SHUTDN_ACHighPrFanSw', '16', '2', 'LE', 'unsigned', 'Standard', '0', '1', '0', '0', '3'; 'ECU_SHUTDN_CoolLvlEngPrShSt', '60', '2', 'LE', 'unsigned', 'Standard', '0', '1', '0', '0', '3'; 'ECU_SHUTDN_EnIdShDAM', '2', '2', 'LE', 'unsigned', 'Standard', '0', '1', '0', '0', '3'; 'ECU_SHUTDN_EnIdShSE', '0', '2', 'LE', 'unsigned', 'Standard', '0', '1', '0', '0', '3'; 'ECU_SHUTDN_EnIdShTF', '14', '2', 'LE', 'unsigned', 'Standard', '0', '1', '0', '0', '3'; 'ECU_SHUTDN_EnIdShTO', '4', '2', 'LE', 'unsigned', 'Standard', '0', '1', '0', '0', '3'; 'ECU_SHUTDN_EnIdShTS', '6', '2', 'LE', 'unsigned', 'Standard', '0', '1', '0', '0', '3'; 'ECU_SHUTDN_EngAirShComSt', '52', '2', 'LE', 'unsigned', 'Standard', '0', '1', '0', '0', '3'; 'ECU_SHUTDN_EngAirShSt', '56', '2', 'LE', 'unsigned', 'Standard', '0', '1', '0', '0', '3'; 'ECU_SHUTDN_EngAlAckn', '48', '2', 'LE', 'unsigned', 'Standard', '0', '1', '0', '0', '3'; 'ECU_SHUTDN_EngAlOutComSt', '50', '2', 'LE', 'unsigned', 'Standard', '0', '1', '0', '0', '3'; 'ECU_SHUTDN_EngOverspTest', '54', '2', 'LE', 'unsigned', 'Standard', '0', '1', '0', '0', '3'; 'ECU_SHUTDN_EngProtSysAppSh', '34', '2', 'LE', 'unsigned', 'Standard', '0', '1', '0', '0', '3'; 'ECU_SHUTDN_EngProtSysConf', '46', '2', 'LE', 'unsigned', 'Standard', '0', '1', '0', '0', '3'; 'ECU_SHUTDN_EngProtSysShEng', '32', '2', 'LE', 'unsigned', 'Standard', '0', '1', '0', '0', '3'; 'ECU_SHUTDN_EngProtSysTimOver', '36', '2', 'LE', 'unsigned', 'Standard', '0', '1', '0', '0', '3'; 'ECU_SHUTDN_EngProtSysTimSt', '38', '2', 'LE', 'unsigned', 'Standard', '0', '1', '0', '0', '3'; 'ECU_SHUTDN_EngWaitStLam', '24', '2', 'LE', 'unsigned', 'Standard', '0', '1', '0', '0', '3'; 'ECU_SHUTDN_PTOShSE', '58', '2', 'LE', 'unsigned', 'Standard', '0', '1', '0', '0', '3'; 'ECU_SHUTDN_RefrHiPrSw', '20', '2', 'LE', 'unsigned', 'Standard', '0', '1', '0', '0', '3'; 'ECU_SHUTDN_RefrLowPrSw', '18', '2', 'LE', 'unsigned', 'Standard', '0', '1', '0', '0', '3' }  IDPort=off  TimestampPort=off  ErrorPort=off  RemotePort=off  LengthPort=off  StatusPort=off  ApplyMinMax=off
  CANUnpack_ECU_VEP1 : canmsglib/CAN Unpack  MsgList=(none)  MsgName=ECU_VEP1  MsgIDType=Extended (29-bit identifier)  MsgIdentifier=419362560  MsgLength=8  SignalInfo={ 'ECU_VEP1_AltCur', '8', '8', 'LE', 'unsigned', 'Standard', '0', '1', '-125', '-125', '125'; 'ECU_VEP1_BatPot', '32', '16', 'LE', 'unsigned', 'Standard', '0', '0.05', '0', '0', '3212.75'; 'ECU_VEP1_ChrgSysPot', '16', '16', 'LE', 'unsigned', 'Standard', '0', '0.05', '0', '0', '3212.75'; 'ECU_VEP1_KeyswPot', '48', '16', 'LE', 'unsigned', 'Standard', '0', '0.05', '0', '0', '3212.75'; 'ECU_VEP1_NetBatCur', '0', '8', 'LE', 'unsigned', 'Standard', '0', '1', '-125', '-125', '125' }  IDPort=off  TimestampPort=off  ErrorPort=off  RemotePort=off  LengthPort=off  StatusPort=off  ApplyMinMax=off
  Data Store Write : DataStoreWrite  DataStoreName=InputNetworkData  DataStoreElements=InputNetworkData.EngCAN.EngTotalHours  IndexOptions=Index vector (dialog)  Indices=1  OutputSizes=1
  Data Store Write1 : DataStoreWrite  DataStoreName=InputNetworkData  DataStoreElements=InputNetworkData.EngCAN.EngAirFiltRestrLampCmd#InputNetworkData.EngCAN.EngAmberWarnLampCmd#InputNetworkData.EngCAN.EngCoolLevLowLampCmd#InputNetworkData.EngCAN.EngCoolTempHiLampCmd#InputNetworkData.EngCAN.EngOilPressLowLampCmd#InputNetworkData.EngCAN.EngProtLampCmd#InputNetworkData.EngCAN.EngRedStopLampCmd  IndexOptions=Index vector (dialog)  Indices=1  OutputSizes=1
  Data Store Write2 : DataStoreWrite  Commented=on  DataStoreName=InputNetworkData  DataStoreElements=InputNetworkData.EngCAN.EngTotalHours  IndexOptions=Index vector (dialog)  Indices=1  OutputSizes=1
  Data Store Write4 : DataStoreWrite  DataStoreName=InputNetworkData  DataStoreElements=InputNetworkData.EngCAN.EngCoolTemp#InputNetworkData.EngCAN.EngFuelTemp1#InputNetworkData.EngCAN.EngIntThOp#InputNetworkData.EngCAN.EngInterTemp#InputNetworkData.EngCAN.EngOilTemp1#InputNetworkData.EngCAN.EngTurbOilTemp  IndexOptions=Index vector (dialog)  Indices=1  OutputSizes=1
  Data Store Write5 : DataStoreWrite  DataStoreName=InputNetworkData  DataStoreElements=InputNetworkData.EngCAN.EngECUTemp#InputNetworkData.EngCAN.EngExGasRec1T#InputNetworkData.EngCAN.EngExhGasRec1DP#InputNetworkData.EngCAN.EngOilTemp2  IndexOptions=Index vector (dialog)  Indices=1  OutputSizes=1
  Data Store Write6 : DataStoreWrite  DataStoreName=InputNetworkData  DataStoreElements=InputNetworkData.EngCAN.ACHighPrFanSw#InputNetworkData.EngCAN.CoolLvlEngPrShSt#InputNetworkData.EngCAN.EnIdShDAM#InputNetworkData.EngCAN.EnIdShSE#InputNetworkData.EngCAN.EnIdShTF#InputNetworkData.EngCAN.EnIdShTO#InputNetworkData.EngCAN.EnIdShTS#InputNetworkData.EngCAN.EngAirShComSt#InputNetworkData.EngCAN.EngAirShSt#InputNetworkData.EngCAN.EngAlAckn#InputNetworkData.EngCAN.EngAlOutComSt#InputNetworkData.EngCAN.EngOverspTest#InputNetworkData.EngCAN.EngProtSysAppSh#InputNetworkData.EngCAN.EngProtSysConf#InputNetworkData.EngCAN.EngProtSysShEng#InputNetworkData.EngCAN.EngProtSysTimOver#InputNetworkData.EngCAN.EngProtSysTimSt#InputNetworkData.EngCAN.EngWaitStLam#InputNetworkData.EngCAN.PTOShSE#InputNetworkData.EngCAN.RefrHiPrSw#InputNetworkData.EngCAN.RefrLowPrSw  IndexOptions=Index vector (dialog)  Indices=1  OutputSizes=1
  Data Store Write7 : DataStoreWrite  DataStoreName=InputNetworkData  DataStoreElements=InputNetworkData.EngCAN.AltCur#InputNetworkData.EngCAN.BatPot#InputNetworkData.EngCAN.ChrgSysPot#InputNetworkData.EngCAN.KeyswPot#InputNetworkData.EngCAN.NetBatCur  IndexOptions=Index vector (dialog)  Indices=1  OutputSizes=1
  Function Caller1 : FunctionCaller  FunctionPrototype=rawValue = convUintPinToenumStt(uintValue)  InputArgumentSpecifications=<Enter example>  OutputArgumentSpecifications=<Enter example>
  MATLAB Function : MATLAB Function  TreatAsAtomicUnit=on
  Terminator{,1..5} (6 alike) : Terminator
  read_DLCC1 : TTlibrary/CAN/read_message_name  channel=IO_CAN_CHANNEL_2  id_format=IO_CAN_EXT_FRAME  get_msg_info=off  message_names=there is no CAN Unpack blocks  message_info=|  id=419235584  ac_mask=536870911  retranslation=off  io_error=on  sample_time=-1
      | Message Name: ECU_VEP1
      |  Message ID Type: Extended (29-bit identifier)
      |  Message ID: 419362560
      settings: SourceProductName=TT control 500 series
  read_DLCC2 : TTlibrary/CAN/read_message_name  channel=IO_CAN_CHANNEL_2  id_format=IO_CAN_EXT_FRAME  get_msg_info=off  message_names=there is no CAN Unpack blocks  message_info=|  id=419357952  ac_mask=536870911  retranslation=off  io_error=on  sample_time=-1
      | Message Name: ECU_VEP1
      |  Message ID Type: Extended (29-bit identifier)
      |  Message ID: 419362560
      settings: SourceProductName=TT control 500 series
  read_ECU_ET1 : TTlibrary/CAN/read_message_name  channel=IO_CAN_CHANNEL_2  id_format=IO_CAN_EXT_FRAME  get_msg_info=off  message_names=there is no CAN Unpack blocks  message_info=|  id=419360256  ac_mask=536870911  retranslation=off  io_error=on  sample_time=-1
      | Message Name: ECU_ET1
      |  Message ID Type: Extended (29-bit identifier)
      |  Message ID: 419360256
      settings: SourceProductName=TT control 500 series
  read_ECU_ET2 : TTlibrary/CAN/read_message_name  channel=IO_CAN_CHANNEL_2  id_format=IO_CAN_EXT_FRAME  get_msg_info=off  message_names=there is no CAN Unpack blocks  message_info=|  id=419341312  ac_mask=536870911  retranslation=off  io_error=on  sample_time=-1
      | Message Name: ECU_ET2
      |  Message ID Type: Extended (29-bit identifier)
      |  Message ID: 419341312
      settings: SourceProductName=TT control 500 series
  read_ECU_SHUTDN : TTlibrary/CAN/read_message_name  channel=IO_CAN_CHANNEL_2  id_format=IO_CAN_EXT_FRAME  get_msg_info=off  message_names=there is no CAN Unpack blocks  message_info=|  id=419357696  ac_mask=536870911  retranslation=off  io_error=on  sample_time=-1
      | Message Name: ECU_SHUTDN
      |  Message ID Type: Extended (29-bit identifier)
      |  Message ID: 419357696
      settings: SourceProductName=TT control 500 series
  read_ECU_VEP1 : TTlibrary/CAN/read_message_name  channel=IO_CAN_CHANNEL_2  id_format=IO_CAN_EXT_FRAME  get_msg_info=off  message_names=there is no CAN Unpack blocks  message_info=|  id=419362560  ac_mask=536870911  retranslation=off  io_error=on  sample_time=-1
      | Message Name: ECU_VEP1
      |  Message ID Type: Extended (29-bit identifier)
      |  Message ID: 419362560
      settings: SourceProductName=TT control 500 series
  wires:
  CANUnpack_ECU_ET3/1 -> Data Store Write/1
  read_DLCC2/2 -> Terminator5/1  "handler_err_419357952"
  read_DLCC2/1 -> CANUnpack_ECU_ET3/1  "msg_419357952"
  CANUnpack_ECU_DLCC1/7 -> Data Store Write1/7
  CANUnpack_ECU_DLCC1/6 -> Data Store Write1/6
  CANUnpack_ECU_DLCC1/5 -> Data Store Write1/5
  CANUnpack_ECU_DLCC1/4 -> Data Store Write1/4
  CANUnpack_ECU_DLCC1/3 -> Data Store Write1/3
  CANUnpack_ECU_DLCC1/2 -> Data Store Write1/2
  CANUnpack_ECU_DLCC1/1 -> Data Store Write1/1
  read_DLCC1/1 -> CANUnpack_ECU_DLCC1/1  "msg_419235584"
  read_DLCC1/2 -> Terminator4/1  "handler_err_419235584"
  MATLAB Function/1(coolLvlState) -> Data Store Write6/2
  CANUnpack_ECU_ET1/5 -> Data Store Write4/5
  Function Caller1/1 -> Data Store Write6/18
  read_ECU_VEP1/2 -> Terminator3/1  "handler_err_419362560"
  read_ECU_SHUTDN/2 -> Terminator2/1  "handler_err_419357696"
  read_ECU_ET2/2 -> Terminator1/1  "handler_err_419341312"
  read_ECU_ET1/2 -> Terminator/1  "handler_err_419360256"
  CANUnpack_ECU_SHUTDN/13 -> Data Store Write6/13
  CANUnpack_ECU_ET1/3 -> Data Store Write4/3
  CANUnpack_ECU_ET2/1 -> Data Store Write5/1
  CANUnpack_ECU_VEP1/2 -> Data Store Write7/2
  CANUnpack_ECU_SHUTDN/1 -> Data Store Write6/1
  CANUnpack_ECU_VEP1/1 -> Data Store Write7/1
  CANUnpack_ECU_ET1/4 -> Data Store Write4/4
  CANUnpack_ECU_SHUTDN/3 -> Data Store Write6/3
  CANUnpack_ECU_VEP1/5 -> Data Store Write7/5
  CANUnpack_ECU_SHUTDN/2 -> MATLAB Function/1(Value)
  CANUnpack_ECU_ET2/2 -> Data Store Write5/2
  CANUnpack_ECU_ET1/2 -> Data Store Write4/2
  CANUnpack_ECU_ET2/3 -> Data Store Write5/3
  CANUnpack_ECU_ET2/4 -> Data Store Write5/4
  CANUnpack_ECU_SHUTDN/5 -> Data Store Write6/5
  CANUnpack_ECU_SHUTDN/6 -> Data Store Write6/6
  CANUnpack_ECU_SHUTDN/8 -> Data Store Write6/8
  CANUnpack_ECU_SHUTDN/16 -> Data Store Write6/16
  CANUnpack_ECU_SHUTDN/9 -> Data Store Write6/9
  CANUnpack_ECU_SHUTDN/11 -> Data Store Write6/11
  CANUnpack_ECU_SHUTDN/10 -> Data Store Write6/10
  CANUnpack_ECU_SHUTDN/14 -> Data Store Write6/14
  CANUnpack_ECU_ET1/6 -> Data Store Write4/6
  CANUnpack_ECU_SHUTDN/15 -> Data Store Write6/15
  CANUnpack_ECU_SHUTDN/18 -> Function Caller1/1
  CANUnpack_ECU_SHUTDN/21 -> Data Store Write6/21
  CANUnpack_ECU_VEP1/3 -> Data Store Write7/3
  CANUnpack_ECU_VEP1/4 -> Data Store Write7/4
  CANUnpack_ECU_ET1/1 -> Data Store Write4/1
  CANUnpack_ECU_SHUTDN/12 -> Data Store Write6/12
  CANUnpack_ECU_SHUTDN/17 -> Data Store Write6/17
  CANUnpack_ECU_SHUTDN/20 -> Data Store Write6/20
  read_ECU_ET1/1 -> CANUnpack_ECU_ET1/1  "msg_419360256"
  read_ECU_SHUTDN/1 -> CANUnpack_ECU_SHUTDN/1  "msg_419357696"
  CANUnpack_ECU_SHUTDN/19 -> Data Store Write6/19
  CANUnpack_ECU_SHUTDN/4 -> Data Store Write6/4
  read_ECU_VEP1/1 -> CANUnpack_ECU_VEP1/1  "msg_419362560"
  CANUnpack_ECU_SHUTDN/7 -> Data Store Write6/7
  read_ECU_ET2/1 -> CANUnpack_ECU_ET2/1  "msg_419341312"
